simulink model "OvervoltageRelayBlock"  (R2016a)
settings: Solver=ode23tb  StartTime=0.0  StopTime=1  RelTol=1e-3
libraries: powerlib x8, powerlib_meascontrol x1
settings Model: Creator=Rodney Tan  LastModifiedBy=Rodney Tan
settings DataIOCC: LimitDataPoints=on  SaveFormat=Array
settings HardwareCC: ProdBitPerPointer=32  ProdLargestAtomicFloat=None  ProdIntDivRoundTo=Undefined  ProdEndianess=Unspecified  ProdWordSize=32  ProdHWDeviceType=32-bit Generic
settings ModelReferenceCC: PropagateSignalLabelsOutOfModel=off
settings ConfigComp: CovModelRefEnable=Off

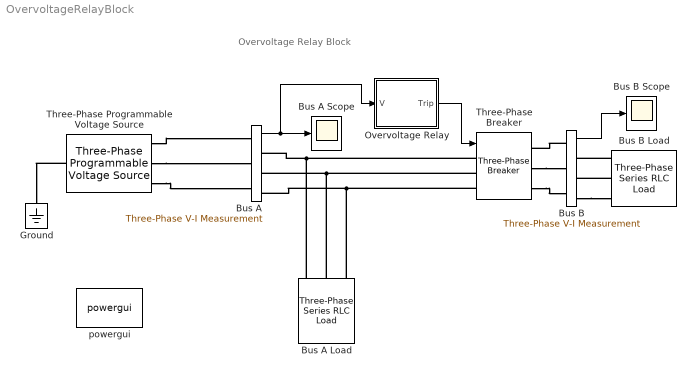
== system OvervoltageRelayBlock ==
  note: Overvoltage Relay Block
  Bus A : powerlib/Measurements/Three-Phase V-I Measurement  VoltageMeasurement=phase-to-ground  SetLabelV=off  LabelV=Vabc  Vpu=off  VpuLL=off  CurrentMeasurement=no  SetLabelI=off  LabelI=Iabc  Ipu=off  Pbase=100e6  Vbase=500e3  OutputType=Complex  PhasorSimulation=off  PSBequivalent=0
  Bus A Load : powerlib/Elements/Three-Phase Series RLC Load  LConnTagsString=A|B|C  Configuration=Y (grounded)  NominalVoltage=400  Vabc=[1e3 1e3 1e3]  Vabcp=[1e3 1e3 1e3]  NominalFrequency=50  UnbalancedPower=off  ActivePower=100e3  InductivePower=1000  CapacitivePower=0  Pabc=[10e3 9e3 11e3]  QLabc=[100 90 110]  QCabc=[100 90 110]  Pabcp=[10e3 9e3 11e3]  QLabcp=[100 90 110]  QCabcp=[100 90 110]  Measurements=None  LoadType=constant Z
  Bus A Scope : Scope
  Bus B : powerlib/Measurements/Three-Phase V-I Measurement  VoltageMeasurement=phase-to-ground  SetLabelV=off  LabelV=Vabc  Vpu=off  VpuLL=off  CurrentMeasurement=no  SetLabelI=off  LabelI=Iabc  Ipu=off  Pbase=100e6  Vbase=500e3  OutputType=Complex  PhasorSimulation=off  PSBequivalent=0
  Bus B Load : powerlib/Elements/Three-Phase Series RLC Load  LConnTagsString=A|B|C  Configuration=Y (grounded)  NominalVoltage=400  Vabc=[1e3 1e3 1e3]  Vabcp=[1e3 1e3 1e3]  NominalFrequency=50  UnbalancedPower=off  ActivePower=100e3  InductivePower=1000  CapacitivePower=0  Pabc=[10e3 9e3 11e3]  QLabc=[100 90 110]  QCabc=[100 90 110]  Pabcp=[10e3 9e3 11e3]  QLabcp=[100 90 110]  QCabcp=[100 90 110]  Measurements=None  LoadType=constant Z
  Bus B Scope : Scope
  Ground : powerlib/Elements/Ground  LConnTagsString=a
  Overvoltage Relay : Subsystem  mask(Over Voltage Relay Block){OVset=10, delay=0.2, Vn=230, Freq=50}
      mask prompts: OVset "Overvoltage Setting (1-25%)"; delay "Overvoltage Ride Through Time Delay (0.1-30s)"; Vn "Nonimal Phase-to-Ground Voltage (Vrms)"; Freq "Fundamental frequency (Hz):"
      mask help:
      | Overvoltage Relay Block developed by Dr. Rodney Tan
      | Version 1.0 (Aug 2017)
      |
      | Overvoltage Relay (ANSI/IEEE C37.2 device number 59) that operates when the voltage exceeds the predetermined value.
      mask Help:
      | <b>Overvoltage Setting  (U <<)</b>
      | Specify overvoltage setting ranging from 1% to 25%.
      | 
      | <b>Overvoltage Time Delay Setting (t <<)</b>
      | Specify overvoltage time delay ranging from 0.1s to 30s for under voltage ride through.
      | 
      | <b>Nominal Phase-to-Ground Voltage (Vrms)</b>
      | Specify the relay nominal phase-to-ground RMS voltage measurement.
      | 
      | <b>Fundamental Frequency (Hz)</b>
      | Specify the RMS current measurement fundamental frequency, in hertz, of the input signal.
      mask Callback OVset:
      | OVset = str2double(get_param(gcb,'OVset'));
      | if (OVset > 25)||(OVset < 1)||isnan(OVset)
      |     msgbox('Over Voltage Setting must be in the range of 1-25%',...
      |     'Invalid Value !','error');
      |     set_param(gcb,'OVset','10');
      | end
      mask Callback delay:
      | delay = str2double(get_param(gcb,'delay'));
      | if (delay > 30)||(delay < 0.1)||isnan(delay)
      |     msgbox('Over Voltage Time Delay Setting must be in the range of 0.1-30s',...
      |     'Invalid Value !','error');
      |     set_param(gcb,'delay','1');
      | end
      mask TypeOptions Freq: Vrms/Freq
      mask DialogControl Container1 Prompt: Voltage Measurement
      mask Display:
      | disp('(59)');
      | port_label('input', 1, 'V');
      | port_label('output', 1, 'Trip');
  Three-Phase Programmable Voltage Source : powerlib/Electrical Sources/Three-Phase Programmable Voltage Source  PositiveSequence="[400  0 50]"  VariationEntity=Amplitude  VariationType=Table of time-amplitude pairs  VariationTypeAlt=Step  VariationStep=0.5  VariationRate=10  VariationMagnitude=0.3  VariationFrequency=2  VariationTiming=[1 2]  VariationPhaseA=off  Amplitudes=[1.0 1.2 1.0]  TimeValues=[0 0.1 0.5]  HarmonicGeneration=off  HarmonicA=[3 0.2 -25 0]  HarmonicB=[2 0.15 35 2]  Timing="[0.05  3]"  BusType=swing  Pref=0  Qref=0  Qmin=-inf  Qmax=inf
  Three-Phase Breaker : powerlib/Elements/Three-Phase Breaker  InitialState=closed  SwitchA=on  SwitchB=on  SwitchC=on  SwitchTimes="[1/60  5/60]"  External=on  BreakerResistance=0.01  SnubberResistance=1e6  SnubberCapacitance=inf  Measurements=None
  powergui : powerlib/powergui  Priority=1  SimulationMode=Continuous  SolverType=Tustin/Backward Euler (TBE)  SampleTime=50e-6  frequency=60  SPID=on  DisableSnubberDevices=on  DisableRonSwitches=off  DisableVfSwitches=off  SwTol=0  DisplayEquations=off  Interpol=off  ExternalGateDelay=off  methode=off  Ts=100  FunctionMessages=off  echomessages=off  HookPort=off  EnableUseOfTLC=off  x0status=blocks  frequencyindice=50  Pbase=100e6  ErrMax=1e-4  Iterations=50  UnitsV=kV  UnitsW=MW  buscounter=0  RestoreLinks=warning  ResistiveCurrentMeasurement=off  Frange=[0:2:500]  Ylog=off  Xlog=on  ShowGrid=off  save=off  variable=ZData  structure=0  ZoomFFT=off  StartTime=0.0  cycles=1  DisplayStyle=1  fundamental=60  FreqAxis=off  MaxFrequency=1000  frequencyindicesteady=1  RmsSteady=1  display=off
  wires:
  Bus A/1 -> Overvoltage Relay/1(V), Bus A Scope/1
  Bus B/1 -> Bus B Scope/1
  Overvoltage Relay/1(Trip) -> Three-Phase Breaker/1
  connections:
  Three-Phase Programmable Voltage Source/RConn1 -- Bus A/LConn1
  Three-Phase Breaker/LConn2 -- Bus A Load/LConn2 -- Bus A/RConn2
  Three-Phase Breaker/LConn1 -- Bus A Load/LConn1 -- Bus A/RConn1
  Three-Phase Programmable Voltage Source/RConn2 -- Bus A/LConn2
  Three-Phase Programmable Voltage Source/RConn3 -- Bus A/LConn3
  Three-Phase Breaker/LConn3 -- Bus A Load/LConn3 -- Bus A/RConn3
  Three-Phase Breaker/RConn2 -- Bus B/LConn2
  Bus B/LConn1 -- Three-Phase Breaker/RConn1
  Three-Phase Breaker/RConn3 -- Bus B/LConn3
  Bus B Load/LConn2 -- Bus B/RConn2
  Bus B/RConn3 -- Bus B Load/LConn3
  Bus B Load/LConn1 -- Bus B/RConn1
  Three-Phase Programmable Voltage Source/LConn1 -- Ground/LConn1

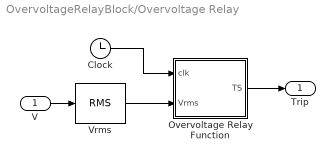
== system OvervoltageRelayBlock/Overvoltage Relay ==
  V : Inport
  Clock : Clock
  Overvoltage Relay Function : MATLAB Function  TreatAsAtomicUnit=on
  Vrms : powerlib_meascontrol/Measurements/RMS  TrueRMS=on  Freq=Freq  RMSInit=0  Ts=0
  Trip : Outport
  wires:
  Clock/1 -> Overvoltage Relay Function/1(clk)
  Vrms/1 -> Overvoltage Relay Function/2(Vrms)
  Overvoltage Relay Function/1(TS) -> Trip/1
  V/1 -> Vrms/1

== matlab function OvervoltageRelayBlock/Overvoltage Relay/Overvoltage Relay Function ==
  data: clk input; TS output; Vrms input; Vn parameter; OVset parameter; delay parameter
function TS = fcn(clk,Vrms,Vn,OVset,delay)

persistent RelayState TripTime CaptureClk StopClk

if isempty(RelayState)
    RelayState = 0;     % Reset Relay
    TripTime = inf;
    CaptureClk = 0;
    StopClk = 0;
end

if max(Vrms)>=(Vn+(Vn*(OVset/100)))
    if (CaptureClk == 0)
        StopClk = clk + delay; % Capture current clock plus delay time
        CaptureClk = 1;
    end
    if (RelayState == 0)&&(clk-StopClk >= 0)
       TripTime = clk + 0.02; % Added 20ms delay due to mechanical relay contact movement
       RelayState = 1;
    end
else
    CaptureClk = 0;
end

TS = (clk <= TripTime);
